simulink model "ES205_lab_5_lower_model_mod"  (R2021a)
settings: Solver=VariableStepAuto  StartTime=0.0  StopTime=tf_lower  MaxStep=maxstep  RelTol=tol  AbsTol=tol
values from neighbouring files (symbols this model uses):
  a2 = 3.24    [ES205_lab_5_script.m]
  Aout2 = pi * (d2/2)^2    (= 0.0452389342117)    [ES205_lab_5_script.m]
  Atank2 = 22.94    [ES205_lab_5_script.m]
  b2 = 0.5    [ES205_lab_5_script.m]
  Cd2_mod = values2(si)    [ES205_lab_5_script.m]
  g = 32.2 * 12    (= 386.4)    [ES205_lab_5_script.m]
  h2_0_single = 9    [ES205_lab_5_script.m]
settings Model: Creator=schimmer  LastModifiedBy=schimmer
settings DataIOCC: SaveOutput=off  SignalLogging=off  DSMLogging=off  SaveTime=off  ReturnWorkspaceOutputs=off  OutputOption=SpecifiedOutputTimes  OutputTimes=tdata_lower

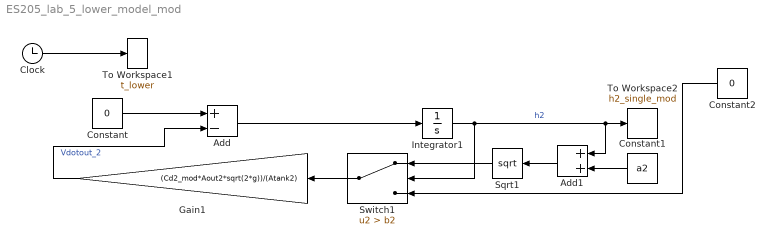
== system ES205_lab_5_lower_model_mod ==
  Add : Sum  Inputs=+-
  Add1 : Sum
  Clock : Clock
  Constant : Constant  Value=0
  Constant1 : Constant  Value=a2
  Constant2 : Constant  Value=0
  Gain1 : Gain  Gain=(Cd2_mod*Aout2*sqrt(2*g))/(Atank2)
  Integrator1 : Integrator  InitialCondition=h2_0_single
  Sqrt1 : Sqrt  SaturateOnIntegerOverflow=on
  Switch1 : Switch  Criteria=u2 > Threshold  Threshold=b2
  To Workspace1 : ToWorkspace  VariableName=t_lower  SampleTime=-1
  To Workspace2 : ToWorkspace  VariableName=h2_single_mod  SampleTime=-1
  wires:
  Clock/1 -> To Workspace1/1
  Constant1/1 -> Add1/2
  Integrator1/1 -> Switch1/2, Add1/1, To Workspace2/1  "h2"
  Add1/1 -> Sqrt1/1
  Sqrt1/1 -> Switch1/1
  Constant2/1 -> Switch1/3
  Switch1/1 -> Gain1/1
  Add/1 -> Integrator1/1
  Constant/1 -> Add/1
  Gain1/1 -> Add/2  "Vdotout_2"
